simulink model "PruebaTakagi"  (R2015a)
settings: Solver=ode45  StartTime=0.0  StopTime=0.032  RelTol=1e-3
libraries: fl_lib x26, nesl_utility x10
settings Model: Creator=NECSOFT  LastModifiedBy=NECSOFT

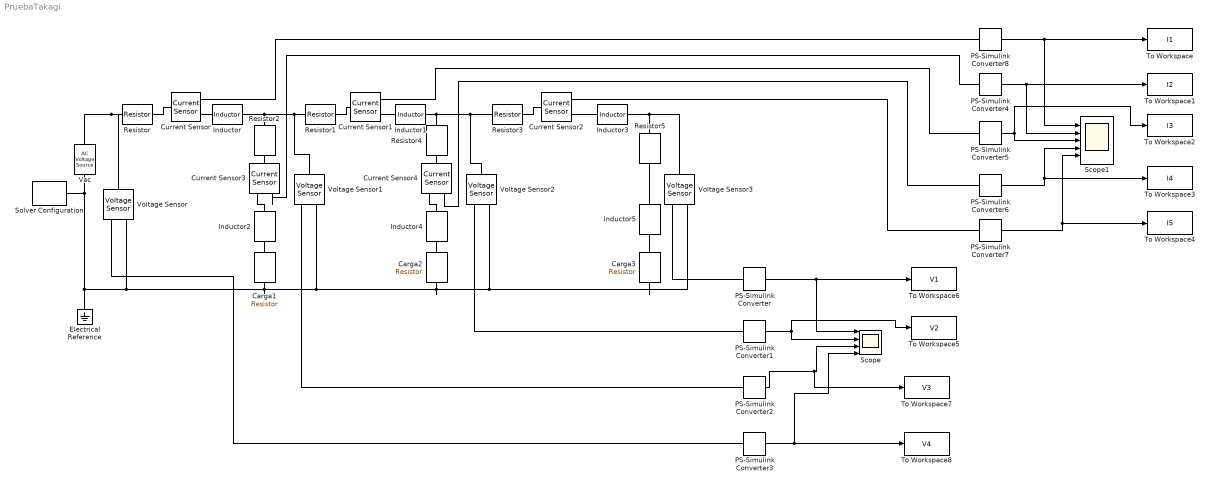
== system PruebaTakagi ==
  Carga1 : fl_lib/Electrical/Electrical Elements/Resistor  R=1 kOhm  i_specify=off  i_priority=High  i=0 A  v_specify=off  v_priority=High  v=0 V
  Carga2 : fl_lib/Electrical/Electrical Elements/Resistor  R=10 kOhm  i_specify=off  i_priority=High  i=0 A  v_specify=off  v_priority=High  v=0 V
  Carga3 : fl_lib/Electrical/Electrical Elements/Resistor  R=0.5 kOhm  i_specify=off  i_priority=High  i=0 A  v_specify=off  v_priority=High  v=0 V
  Current Sensor{,1..4} (5 alike) : fl_lib/Electrical/Electrical Sensors/Current Sensor
  Electrical Reference : fl_lib/Electrical/Electrical Elements/Electrical Reference
  Inductor : fl_lib/Electrical/Electrical Elements/Inductor  l=1e-3 H  r=0 Ohm  g=1e-9 1/Ohm  i_specify=off  i_priority=High  i=0 A  v_specify=off  v_priority=High  v=0 V  i_L_specify=off  i_L_priority=High  i_L=0 A
  Inductor1 : fl_lib/Electrical/Electrical Elements/Inductor  l=3e-3 H  r=0 Ohm  g=1e-9 1/Ohm  i_specify=off  i_priority=High  i=0 A  v_specify=off  v_priority=High  v=0 V  i_L_specify=off  i_L_priority=High  i_L=0 A
  Inductor2 : fl_lib/Electrical/Electrical Elements/Inductor  l=2e-3 H  r=0 Ohm  g=1e-9 1/Ohm  i_specify=off  i_priority=High  i=0 A  v_specify=off  v_priority=High  v=0 V  i_L_specify=off  i_L_priority=High  i_L=0 A
  Inductor3 : fl_lib/Electrical/Electrical Elements/Inductor  l=6e-3 H  r=0 Ohm  g=1e-9 1/Ohm  i_specify=off  i_priority=High  i=0 A  v_specify=off  v_priority=High  v=0 V  i_L_specify=off  i_L_priority=High  i_L=0 A
  Inductor4 : fl_lib/Electrical/Electrical Elements/Inductor  l=5e-3 H  r=0 Ohm  g=1e-9 1/Ohm  i_specify=off  i_priority=High  i=0 A  v_specify=off  v_priority=High  v=0 V  i_L_specify=off  i_L_priority=High  i_L=0 A
  Inductor5 : fl_lib/Electrical/Electrical Elements/Inductor  l=6e-3 H  r=0 Ohm  g=1e-9 1/Ohm  i_specify=off  i_priority=High  i=0 A  v_specify=off  v_priority=High  v=0 V  i_L_specify=off  i_L_priority=High  i_L=0 A
  PS-Simulink Converter{,1..8} (9 alike) : nesl_utility/PS-Simulink Converter  PhysicalDomain=network_engine_domain  SubClassName=ps_output  LeftPortType=input  RightPortType=output  PseudoPeriodic=off  Frequencies=[]  Unit=1  AffineConversion=off
  Resistor : fl_lib/Electrical/Electrical Elements/Resistor  R=1 Ohm  i_specify=off  i_priority=High  i=0 A  v_specify=off  v_priority=High  v=0 V
  Resistor1 : fl_lib/Electrical/Electrical Elements/Resistor  R=3 Ohm  i_specify=off  i_priority=High  i=0 A  v_specify=off  v_priority=High  v=0 V
  Resistor2 : fl_lib/Electrical/Electrical Elements/Resistor  R=2 Ohm  i_specify=off  i_priority=High  i=0 A  v_specify=off  v_priority=High  v=0 V
  Resistor3 : fl_lib/Electrical/Electrical Elements/Resistor  R=6 Ohm  i_specify=off  i_priority=High  i=0 A  v_specify=off  v_priority=High  v=0 V
  Resistor4 : fl_lib/Electrical/Electrical Elements/Resistor  R=4 Ohm  i_specify=off  i_priority=High  i=0 A  v_specify=off  v_priority=High  v=0 V
  Resistor5 : fl_lib/Electrical/Electrical Elements/Resistor  R=6 Ohm  i_specify=off  i_priority=High  i=0 A  v_specify=off  v_priority=High  v=0 V
  Scope : Scope  NumInputPorts=4
      settings: YMin=-5~-5~-5~-5  YMax=5~5~5~5
  Scope1 : Scope  NumInputPorts=5
      settings: YMin=-0.035~-0.035~-0.035~-0.035~-0.035  YMax=0.035~0.035~0.035~0.035~0.035  ScrollMode=on
  Solver Configuration : nesl_utility/Solver Configuration  PhysicalDomain=network_engine_domain  SubClassName=solver  LeftPortType=input  RightPortType=generic  Accelerate=off  Tones=[]  Harmonics=[]  SimulateNoise=off  Profile=off  UseLocalSampling=off  EnableSwitchedLinearOptims=on  FrequencyDomain=off  UseCCode=off  RelTol=0.001  AbsTol=1e-06  MinStep=1e-09  ToWorkspace=off  RevertToSquareIcSolve=off  NumHomotopyIterations=100  DoDC=off  ResidualTolerance=1e-09  UseLocalSolver=on  LocalSolverChoice=NE_BACKWARD_EULER_ADVANCER  LocalSolverSampleTime=0.0001  DoFixedCost=on  MaxNonlinIter=3  MaxModeIter=2  LinearAlgebra=Sparse  DelaysMemoryBudget=1024  AutomaticFiltering=on  FilteringTimeConstant=0.001
  To Workspace : ToWorkspace  VariableName=I1  SampleTime=-1
  To Workspace1 : ToWorkspace  VariableName=I2  SampleTime=-1
  To Workspace2 : ToWorkspace  VariableName=I3  SampleTime=-1
  To Workspace3 : ToWorkspace  VariableName=I4  SampleTime=-1
  To Workspace4 : ToWorkspace  VariableName=I5  SampleTime=-1
  To Workspace5 : ToWorkspace  VariableName=V2  SampleTime=-1
  To Workspace6 : ToWorkspace  VariableName=V1  SampleTime=-1
  To Workspace7 : ToWorkspace  VariableName=V3  SampleTime=-1
  To Workspace8 : ToWorkspace  VariableName=V4  SampleTime=-1
  Vac : fl_lib/Electrical/Electrical Sources/AC Voltage Source  amp=10 V  shift=0 deg  frequency=60 Hz  omega=0 rad/s
  Voltage Sensor{,1..3} (4 alike) : fl_lib/Electrical/Electrical Sensors/Voltage Sensor
  wires:
  PS-Simulink Converter/1 -> To Workspace6/1, Scope/1
  PS-Simulink Converter1/1 -> Scope/2, To Workspace5/1
  PS-Simulink Converter2/1 -> To Workspace7/1, Scope/3
  PS-Simulink Converter3/1 -> To Workspace8/1, Scope/4
  PS-Simulink Converter8/1 -> To Workspace/1, Scope1/1
  PS-Simulink Converter4/1 -> To Workspace1/1, Scope1/2
  PS-Simulink Converter5/1 -> To Workspace2/1, Scope1/3
  PS-Simulink Converter6/1 -> To Workspace3/1, Scope1/4
  PS-Simulink Converter7/1 -> To Workspace4/1, Scope1/5
  connections:
  Vac/LConn1 -- Voltage Sensor/LConn1 -- Resistor/LConn1
  Electrical Reference/LConn1 -- Solver Configuration/RConn1 -- Vac/RConn1 -- Carga3/RConn1 -- Voltage Sensor3/RConn2 -- Voltage Sensor2/RConn2 -- Carga2/RConn1 -- Voltage Sensor1/RConn2 -- Carga1/RConn1 -- Voltage Sensor/RConn2
  Resistor1/LConn1 -- Resistor2/LConn1 -- Inductor/RConn1 -- Voltage Sensor1/LConn1
  Inductor1/RConn1 -- Resistor4/LConn1 -- Voltage Sensor2/LConn1 -- Resistor3/LConn1
  Resistor5/RConn1 -- Inductor5/LConn1
  Inductor3/RConn1 -- Voltage Sensor3/LConn1 -- Resistor5/LConn1
  Voltage Sensor3/RConn1 -- PS-Simulink Converter/LConn1
  Voltage Sensor2/RConn1 -- PS-Simulink Converter1/LConn1
  Voltage Sensor1/RConn1 -- PS-Simulink Converter2/LConn1
  Voltage Sensor/RConn1 -- PS-Simulink Converter3/LConn1
  Current Sensor/RConn2 -- Inductor/LConn1
  Resistor/RConn1 -- Current Sensor/LConn1
  Carga1/LConn1 -- Inductor2/RConn1
  Inductor4/RConn1 -- Carga2/LConn1
  Carga3/LConn1 -- Inductor5/RConn1
  Current Sensor1/RConn2 -- Inductor1/LConn1
  Resistor1/RConn1 -- Current Sensor1/LConn1
  Current Sensor2/RConn2 -- Inductor3/LConn1
  Resistor3/RConn1 -- Current Sensor2/LConn1
  Current Sensor3/LConn1 -- Resistor2/RConn1
  Current Sensor3/RConn2 -- Inductor2/LConn1
  Current Sensor4/LConn1 -- Resistor4/RConn1
  Current Sensor4/RConn2 -- Inductor4/LConn1
  Current Sensor/RConn1 -- PS-Simulink Converter8/LConn1
  Current Sensor3/RConn1 -- PS-Simulink Converter4/LConn1
  Current Sensor1/RConn1 -- PS-Simulink Converter5/LConn1
  Current Sensor4/RConn1 -- PS-Simulink Converter6/LConn1
  Current Sensor2/RConn1 -- PS-Simulink Converter7/LConn1
